simulink model "RLSimulinkP2PSimul"  (R2021a)
settings: Solver=VariableStepAuto  StartTime=0.0  StopTime=200  RelTol=1e-3
model workspace (MAT data in the model file):
  Sig = Simulink.Signal
  Sig.DataType = 'auto'
  Sig.Dimensions = -1
  Sig.DimensionsMode = 'auto'
  Sig.Complexity = 'auto'
  Sig.SampleTime = -1
  Sig.SamplingMode = 'auto'
undefined symbols (not defined in the file or in its folder): goalPose, speedMax, startPose, steeringRange
libraries: rllib x1
settings Model: OrderedModelArguments=off  Creator=The MathWorks, Inc.  LastModifiedBy=guyot
settings SolverCC: AlgebraicLoopSolver=TrustRegion
settings DebuggingCC: SymbolicDimsDataTypeCodeGenerationDiagnostic=none  SFMachineParentedDataDiag=warning

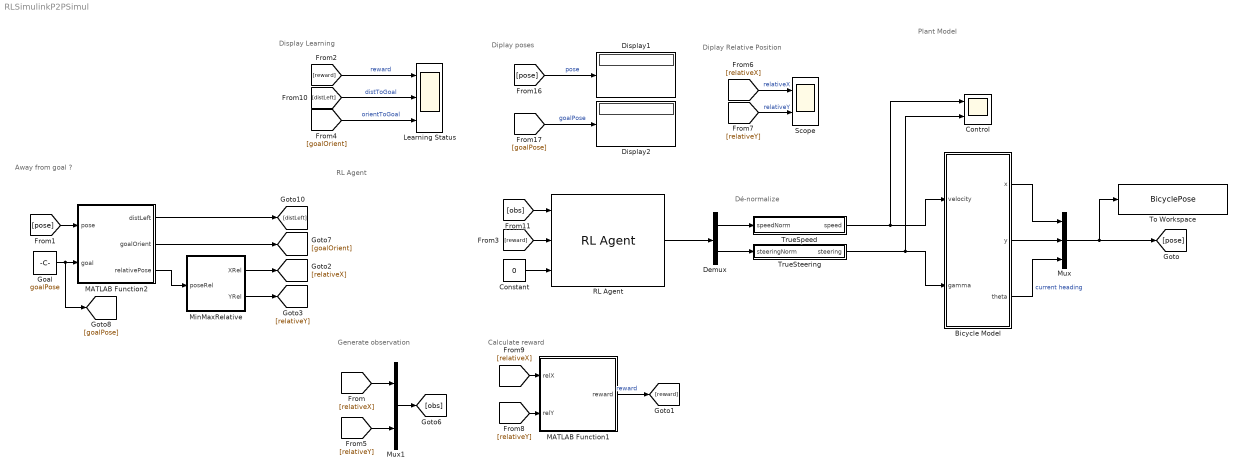
== system RLSimulinkP2PSimul ==
  note: Diplay Relative Position
  note: Diplay poses
  note: Calculate reward
  note: Generate observation
  note: Away from goal ?
  note: Display Learning
  note: RL Agent
  note: Dé-normalize
  note: Plant Model
  Bicycle Model : Subsystem
  Constant : Constant  Value=0
  Control : Scope  NumInputPorts=2
  Demux : Demux  Outputs=2
  Display1 : Display
  Display2 : Display
  Goal : Constant  Value=goalPose
  Learning Status : Scope  NumInputPorts=3
  MATLAB Function1 : MATLAB Function  TreatAsAtomicUnit=on
  MATLAB Function2 : MATLAB Function  TreatAsAtomicUnit=on
  MinMaxRelative : Subsystem
  Mux : Mux  Inputs=3
  Mux1 : Mux  Inputs=2
  RL Agent : rllib/RL Agent  Agent=agent  ExternalActionAsInput=off  ProvideCumRwd=off  TreatAsDirectFeedthrough=on
  Scope : Scope  NumInputPorts=2
  To Workspace : ToWorkspace  VariableName=BicyclePose  SampleTime=-1
  TrueSpeed : Subsystem
  TrueSteering : Subsystem
  wires:
  Mux/1 -> To Workspace/1, [pose]
  RL Agent/1 -> Demux/1
  MATLAB Function1/1(reward) -> [reward]  "reward"
  Bicycle Model/3(theta) -> Mux/3  "current heading"
  Bicycle Model/2(y) -> Mux/2
  Bicycle Model/1(x) -> Mux/1
  TrueSpeed/1(speed) -> Bicycle Model/1(velocity), Control/1
  Demux/2 -> TrueSteering/1(steeringNorm)
  TrueSteering/1(steering) -> Bicycle Model/2(gamma), Control/2
  Demux/1 -> TrueSpeed/1(speedNorm)
  [obs] -> RL Agent/1
  Goal/1 -> [goalPose], MATLAB Function2/2(goal)
  [pose] -> MATLAB Function2/1(pose)
  [reward] -> Learning Status/1  "reward"
  [reward] -> RL Agent/2
  [relativeX] -> MATLAB Function1/1(relX)
  [distLeft] -> Learning Status/2  "distToGoal"
  Mux1/1 -> [obs]
  [relativeX] -> Mux1/1
  [relativeY] -> Mux1/2
  [pose] -> Display1/1  "pose"
  [goalPose] -> Display2/1  "goalPose"
  MATLAB Function2/1(distLeft) -> [distLeft]
  Constant/1 -> RL Agent/3
  [goalOrient] -> Learning Status/3  "orientToGoal"
  MATLAB Function2/2(goalOrient) -> [goalOrient]
  MATLAB Function2/3(relativePose) -> MinMaxRelative/1(poseRel)
  MinMaxRelative/1(XRel) -> [relativeX]
  MinMaxRelative/2(YRel) -> [relativeY]
  [relativeX] -> Scope/1  "relativeX"
  [relativeY] -> Scope/2  "relativeY"
  [relativeY] -> MATLAB Function1/2(relY)

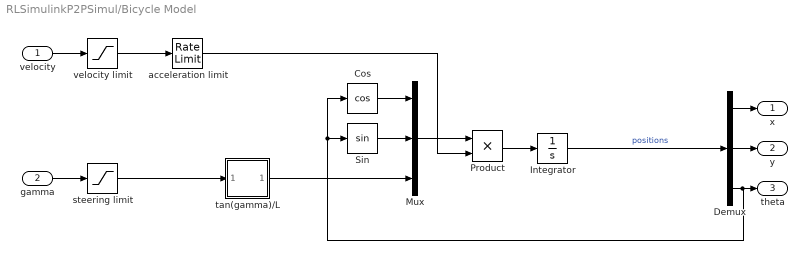
== system RLSimulinkP2PSimul/Bicycle Model ==
  velocity : Inport
  gamma : Inport  Port=2
  Cos : Trigonometry  Operator=cos
  Demux : Demux  Outputs=3
  Integrator : Integrator  InitialCondition=startPose
  Mux : Mux  Inputs=3
  Product : Product
  Sin : Trigonometry
  acceleration limit : RateLimiter  RisingSlewLimit=0.2  SampleTimeMode=inherited
  steering limit : Saturate  UpperLimit=steeringRange  LowerLimit=-steeringRange
  tan(gamma)/L : Subsystem
  velocity limit : Saturate  UpperLimit=speedMax  LowerLimit=-speedMax
  x : Outport
  y : Outport  Port=2
  theta : Outport  Port=3
  wires:
  velocity/1 -> velocity limit/1
  velocity limit/1 -> acceleration limit/1
  gamma/1 -> steering limit/1
  steering limit/1 -> tan(gamma)/L/1(In1)
  tan(gamma)/L/1(Out1) -> Mux/3
  Mux/1 -> Product/1
  acceleration limit/1 -> Product/2
  Product/1 -> Integrator/1
  Integrator/1 -> Demux/1  "positions"
  Demux/3 -> Cos/1, Sin/1, theta/1
  Demux/1 -> x/1
  Demux/2 -> y/1
  Cos/1 -> Mux/1
  Sin/1 -> Mux/2

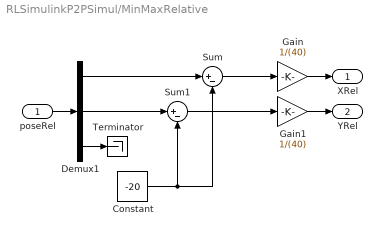
== system RLSimulinkP2PSimul/MinMaxRelative ==
  poseRel : Inport
  Constant : Constant  Value=-20
  Demux1 : Demux  Outputs=3
  Gain : Gain  Gain=1/(40)
  Gain1 : Gain  Gain=1/(40)
  Sum : Sum  Inputs=|+-
  Sum1 : Sum  Inputs=|+-
  Terminator : Terminator
  XRel : Outport
  YRel : Outport  Port=2
  wires:
  Demux1/3 -> Terminator/1
  poseRel/1 -> Demux1/1
  Demux1/2 -> Sum1/1
  Demux1/1 -> Sum/1
  Constant/1 -> Sum1/2, Sum/2
  Sum/1 -> Gain/1
  Sum1/1 -> Gain1/1
  Gain/1 -> XRel/1
  Gain1/1 -> YRel/1

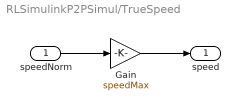
== system RLSimulinkP2PSimul/TrueSpeed ==
  speedNorm : Inport
  Gain : Gain  Gain=speedMax
  speed : Outport
  wires:
  Gain/1 -> speed/1
  speedNorm/1 -> Gain/1

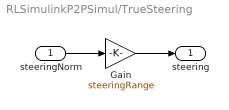
== system RLSimulinkP2PSimul/TrueSteering ==
  steeringNorm : Inport
  Gain : Gain  Gain=steeringRange
  steering : Outport
  wires:
  steeringNorm/1 -> Gain/1
  Gain/1 -> steering/1

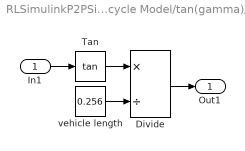
== system RLSimulinkP2PSimul/Bicycle Model/tan(gamma)//L ==
  In1 : Inport
  Divide : Product  Inputs=*/
  Tan : Trigonometry  Operator=tan
  vehicle length : Constant  Value=0.256
  Out1 : Outport
  wires:
  Tan/1 -> Divide/1
  vehicle length/1 -> Divide/2
  In1/1 -> Tan/1
  Divide/1 -> Out1/1

== matlab function RLSimulinkP2PSimul/MATLAB Function1 ==
  data: reward output; relX input; relY input
function reward = calcRew(relX, relY)
    % Fonction de calcul de recompense
    
    % 0.5 < distLeft < sqrt(20^2 + 20^2)
    offset = 0.1 / 40;
    if (relX > 0.5-offset) && (relX < 0.5+offset) && (relY > 0.5-offset) && (relY < 0.5+offset)
        % Arrivé au point : récompense
        reward = 5;
    elseif ((relX > 0.5-offset) && (relX < 0.5+offset)) || ((relY > 0.5-offset) &&(relY < 0.5+offset))
        % Pas encore arrivé : favoriser rapprochement sur un des axes
        reward = 2;
    else
        reward = 0;
    end

== matlab function RLSimulinkP2PSimul/MATLAB Function2 ==
  data: pose input; distLeft output; goal input; goalOrient output; relativePose output
function [distLeft, goalOrient, relativePose] = goalDiff(pose, goal)
    relativePose = goal - pose;

distLeft = sqrt(relativePose(1).^2+relativePose(2).^2);
goalOrient = atan2(relativePose(2),relativePose(1));
